simulink model "quadricopter"  (Simulink 7.4)
settings: Solver=ode45  StartTime=0.0  StopTime=2  RelTol=1e-5
values from neighbouring files (symbols this model uses):
  bm = 5106.8    [PID_init.m]    (also in quad_init.m)
  d = 0.16    [PID_init.m]    (also in quad_init.m)
  g = 9.8    [PID_init.m]    (also in quad_init.m)
  J_x = 7.8*10^-3    (= 0.0078)    [PID_init.m]    (also in quad_init.m)
  J_y = 7.8*10^-3    (= 0.0078)    [PID_init.m]    (also in quad_init.m)
  J_z = 10.22*10^-3    (= 0.01022)    [PID_init.m]    (also in quad_init.m)
  km = 342.4    [PID_init.m]    (also in quad_init.m)
  m = 0.835    [PID_init.m]    (also in quad_init.m)
libraries: aerolibtransform2 x1
settings Model: Creator=diogo  LastModifiedBy=diogo

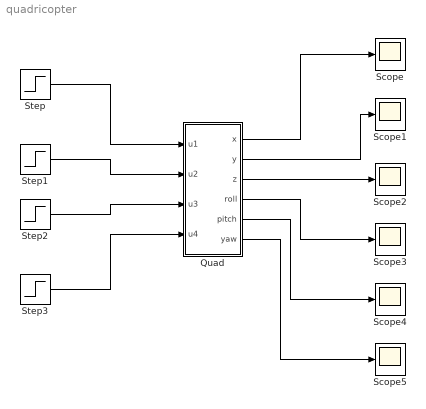
== system quadricopter ==
  Quad : Subsystem
  Scope{,1..5} (6 alike) : Scope
      Scope2 settings: TimeRange=0.03999999999999981  YMin=0  YMax=2e+223  SaveName=ScopeData2
      Scope3 settings: SaveName=ScopeData3
      Scope4 settings: SaveName=ScopeData4
      Scope5 settings: SaveName=ScopeData5
  Step{,1..3} (4 alike) : Step  Time=0  After=0.005  SampleTime=0
  wires:
  Quad/1(x) -> Scope/1
  Quad/2(y) -> Scope1/1
  Quad/3(z) -> Scope2/1
  Quad/4(roll) -> Scope3/1
  Quad/5(pitch) -> Scope4/1
  Quad/6(yaw) -> Scope5/1
  Step/1 -> Quad/1(u1)
  Step1/1 -> Quad/2(u2)
  Step2/1 -> Quad/3(u3)
  Step3/1 -> Quad/4(u4)

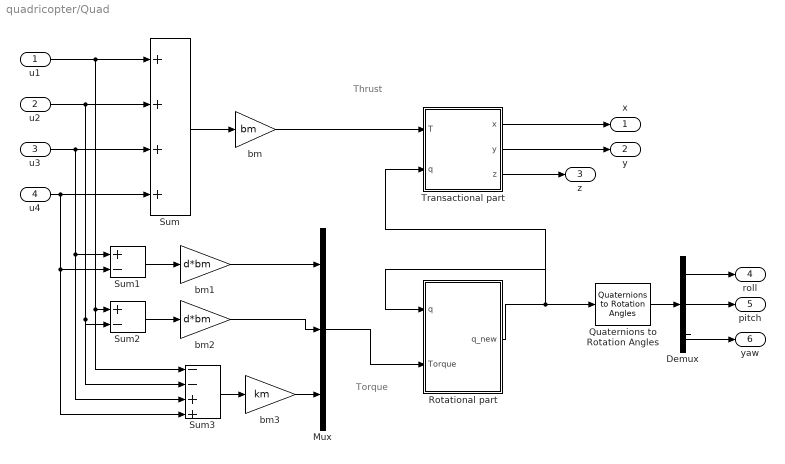
== system quadricopter/Quad ==
  note: Thrust
  note: Torque
  u1 : Inport  OutDataType=fixdt(1, 16)  OutScaling=2^0
  u2 : Inport  Port=2  OutDataType=fixdt(1, 16)  OutScaling=2^0
  u3 : Inport  Port=3  OutDataType=fixdt(1, 16)  OutScaling=2^0
  u4 : Inport  Port=4  OutDataType=fixdt(1, 16)  OutScaling=2^0
  Demux : Demux  Outputs=3
  Mux : Mux  Inputs=3
  Quaternions to Rotation Angles : aerolibtransform2/Quaternions to Rotation Angles  SystemSampleTime=-1  rotationOrder=XYZ
  Rotational part : Subsystem
  Sum : Sum  Inputs=++++  OutDataType=fixdt(1, 16)  OutScaling=2^0
  Sum1 : Sum  Inputs=+-  OutDataType=fixdt(1, 16)  OutScaling=2^0
  Sum2 : Sum  Inputs=+-  OutDataType=fixdt(1, 16)  OutScaling=2^0
  Sum3 : Sum  Inputs=--++  OutDataType=fixdt(1, 16)  OutScaling=2^0
  Transactional part : Subsystem
  bm : Gain  Gain=bm  ParameterDataType=fixdt(1, 16)  ParameterScaling=2^0  OutDataType=fixdt(1, 16)  OutScaling=2^0
  bm1 : Gain  Gain=d*bm  ParameterDataType=fixdt(1, 16)  ParameterScaling=2^0  OutDataType=fixdt(1, 16)  OutScaling=2^0
  bm2 : Gain  Gain=d*bm  ParameterDataType=fixdt(1, 16)  ParameterScaling=2^0  OutDataType=fixdt(1, 16)  OutScaling=2^0
  bm3 : Gain  Gain=km  ParameterDataType=fixdt(1, 16)  ParameterScaling=2^0  OutDataType=fixdt(1, 16)  OutScaling=2^0
  x : Outport  OutDataType=fixdt(1, 16)  OutScaling=2^0
  y : Outport  Port=2  OutDataType=fixdt(1, 16)  OutScaling=2^0
  z : Outport  Port=3  OutDataType=fixdt(1, 16)  OutScaling=2^0
  roll : Outport  Port=4  OutDataType=fixdt(1, 16)  OutScaling=2^0
  pitch : Outport  Port=5  OutDataType=fixdt(1, 16)  OutScaling=2^0
  yaw : Outport  Port=6  OutDataType=fixdt(1, 16)  OutScaling=2^0
  wires:
  u1/1 -> Sum/1, Sum2/1, Sum3/1
  u2/1 -> Sum/2, Sum2/2, Sum3/2
  u3/1 -> Sum/3, Sum1/1, Sum3/3
  u4/1 -> Sum/4, Sum1/2, Sum3/4
  Sum/1 -> bm/1
  bm/1 -> Transactional part/1(T)
  Transactional part/3(z) -> z/1
  Transactional part/2(y) -> y/1
  Transactional part/1(x) -> x/1
  Demux/1 -> roll/1
  Demux/2 -> pitch/1
  Demux/3 -> yaw/1
  Rotational part/1(q_new) -> Transactional part/2(q), Rotational part/1(q), Quaternions to Rotation Angles/1
  Sum1/1 -> bm1/1
  bm1/1 -> Mux/1
  Sum2/1 -> bm2/1
  bm2/1 -> Mux/2
  bm3/1 -> Mux/3
  Sum3/1 -> bm3/1
  Mux/1 -> Rotational part/2(Torque)
  Quaternions to Rotation Angles/1 -> Demux/1

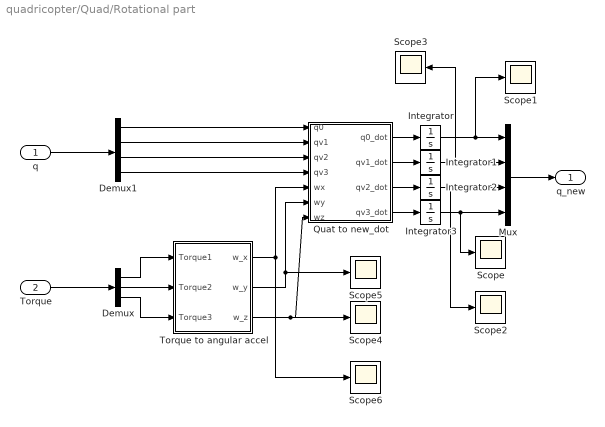
== system quadricopter/Quad/Rotational part ==
  q : Inport  OutDataType=fixdt(1, 16)  OutScaling=2^0
  Torque : Inport  Port=2  OutDataType=fixdt(1, 16)  OutScaling=2^0
  Demux : Demux  Outputs=3
  Demux1 : Demux
  Integrator : Integrator  InitialCondition=1
  Integrator1 : Integrator
  Integrator2 : Integrator
  Integrator3 : Integrator
  Mux : Mux
  Quat to new_dot : Subsystem
  Scope{,1..6} (7 alike) : Scope
      Scope settings: SaveName=ScopeData9
      Scope1 settings: SaveName=ScopeData10
      Scope2 settings: SaveName=ScopeData11
      Scope3 settings: SaveName=ScopeData12
      Scope4 settings: SaveName=ScopeData13
      Scope5 settings: SaveName=ScopeData14
      Scope6 settings: SaveName=ScopeData15
  Torque to angular accel : Subsystem
  q_new : Outport  OutDataType=fixdt(1, 16)  OutScaling=2^0
  wires:
  q/1 -> Demux1/1
  Demux1/1 -> Quat to new_dot/1(q0)
  Demux1/2 -> Quat to new_dot/2(qv1)
  Demux1/3 -> Quat to new_dot/3(qv2)
  Demux1/4 -> Quat to new_dot/4(qv3)
  Torque/1 -> Demux/1
  Demux/1 -> Torque to angular accel/1(Torque1)
  Demux/2 -> Torque to angular accel/2(Torque2)
  Demux/3 -> Torque to angular accel/3(Torque3)
  Torque to angular accel/1(w_x) -> Quat to new_dot/5(wx), Scope6/1
  Torque to angular accel/2(w_y) -> Quat to new_dot/6(wy), Scope5/1
  Torque to angular accel/3(w_z) -> Quat to new_dot/7(wz), Scope4/1
  Quat to new_dot/1(q0_dot) -> Integrator/1
  Quat to new_dot/2(qv1_dot) -> Integrator1/1
  Quat to new_dot/3(qv2_dot) -> Integrator2/1
  Quat to new_dot/4(qv3_dot) -> Integrator3/1
  Integrator/1 -> Mux/1, Scope1/1
  Integrator1/1 -> Mux/2, Scope3/1
  Integrator2/1 -> Mux/3, Scope2/1
  Integrator3/1 -> Mux/4, Scope/1
  Mux/1 -> q_new/1

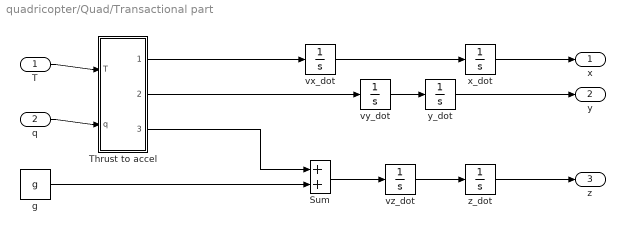
== system quadricopter/Quad/Transactional part ==
  T : Inport  OutDataType=fixdt(1, 16)  OutScaling=2^0
  q : Inport  Port=2  OutDataType=fixdt(1, 16)  OutScaling=2^0
  Sum : Sum  OutDataType=fixdt(1, 16)  OutScaling=2^0
  Thrust to accel : Subsystem
  g : Constant  Value=g  OutDataType=fixdt(1, 16)  OutScaling=2^0
  vx_dot : Integrator
  vy_dot : Integrator
  vz_dot : Integrator
  x_dot : Integrator
  y_dot : Integrator
  z_dot : Integrator
  x : Outport  OutDataType=fixdt(1, 16)  OutScaling=2^0
  y : Outport  Port=2  OutDataType=fixdt(1, 16)  OutScaling=2^0
  z : Outport  Port=3  OutDataType=fixdt(1, 16)  OutScaling=2^0
  wires:
  x_dot/1 -> x/1
  y_dot/1 -> y/1
  z_dot/1 -> z/1
  g/1 -> Sum/2
  T/1 -> Thrust to accel/1(T)
  q/1 -> Thrust to accel/2(q)
  Thrust to accel/1(vx_dot) -> vx_dot/1
  Thrust to accel/2(vy_dot) -> vy_dot/1
  Thrust to accel/3(vz_dot) -> Sum/1
  vz_dot/1 -> z_dot/1
  vy_dot/1 -> y_dot/1
  vx_dot/1 -> x_dot/1
  Sum/1 -> vz_dot/1

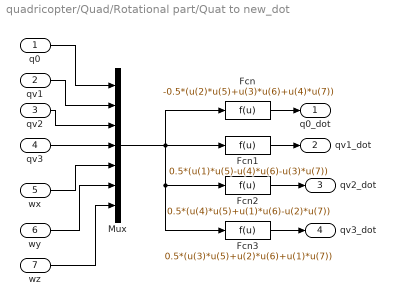
== system quadricopter/Quad/Rotational part/Quat to new_dot ==
  q0 : Inport  OutDataType=fixdt(1, 16)  OutScaling=2^0
  qv1 : Inport  Port=2  OutDataType=fixdt(1, 16)  OutScaling=2^0
  qv2 : Inport  Port=3  OutDataType=fixdt(1, 16)  OutScaling=2^0
  qv3 : Inport  Port=4  OutDataType=fixdt(1, 16)  OutScaling=2^0
  wx : Inport  Port=5  OutDataType=fixdt(1, 16)  OutScaling=2^0
  wy : Inport  Port=6  OutDataType=fixdt(1, 16)  OutScaling=2^0
  wz : Inport  Port=7  OutDataType=fixdt(1, 16)  OutScaling=2^0
  Fcn : Fcn  Expr=-0.5*(u(2)*u(5)+u(3)*u(6)+u(4)*u(7))
  Fcn1 : Fcn  Expr=0.5*(u(1)*u(5)-u(4)*u(6)-u(3)*u(7))
  Fcn2 : Fcn  Expr=0.5*(u(4)*u(5)+u(1)*u(6)-u(2)*u(7))
  Fcn3 : Fcn  Expr=0.5*(u(3)*u(5)+u(2)*u(6)+u(1)*u(7))
  Mux : Mux  Inputs=7
  q0_dot : Outport  OutDataType=fixdt(1, 16)  OutScaling=2^0
  qv1_dot : Outport  Port=2  OutDataType=fixdt(1, 16)  OutScaling=2^0
  qv2_dot : Outport  Port=3  OutDataType=fixdt(1, 16)  OutScaling=2^0
  qv3_dot : Outport  Port=4  OutDataType=fixdt(1, 16)  OutScaling=2^0
  wires:
  q0/1 -> Mux/1
  qv1/1 -> Mux/2
  qv2/1 -> Mux/3
  qv3/1 -> Mux/4
  wx/1 -> Mux/5
  wy/1 -> Mux/6
  wz/1 -> Mux/7
  Mux/1 -> Fcn/1, Fcn1/1, Fcn2/1, Fcn3/1
  Fcn/1 -> q0_dot/1
  Fcn1/1 -> qv1_dot/1
  Fcn2/1 -> qv2_dot/1
  Fcn3/1 -> qv3_dot/1

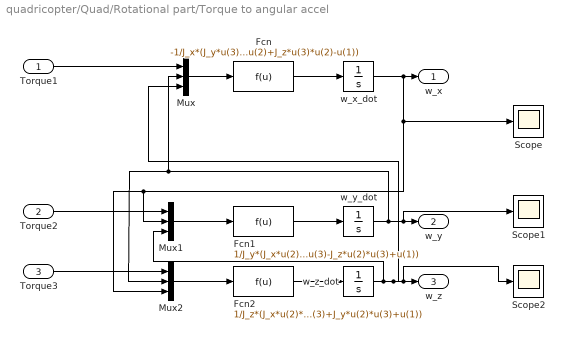
== system quadricopter/Quad/Rotational part/Torque to angular accel ==
  Torque1 : Inport  OutDataType=fixdt(1, 16)  OutScaling=2^0
  Torque2 : Inport  Port=2  OutDataType=fixdt(1, 16)  OutScaling=2^0
  Torque3 : Inport  Port=3  OutDataType=fixdt(1, 16)  OutScaling=2^0
  Fcn : Fcn  Expr=-1/J_x*(J_y*u(3)*u(2)+J_z*u(3)*u(2)-u(1))
  Fcn1 : Fcn  Expr=1/J_y*(J_x*u(2)*u(3)-J_z*u(2)*u(3)+u(1))
  Fcn2 : Fcn  Expr=1/J_z*(J_x*u(2)*u(3)+J_y*u(2)*u(3)+u(1))
  Mux : Mux  Inputs=3
  Mux1 : Mux  Inputs=3
  Mux2 : Mux  Inputs=3
  Scope : Scope
      settings: SaveName=ScopeData6
  Scope1 : Scope
      settings: SaveName=ScopeData7
  Scope2 : Scope
      settings: SaveName=ScopeData8
  w_x_dot : Integrator
  w_y_dot : Integrator
  w_z_dot : Integrator
  w_x : Outport  OutDataType=fixdt(1, 16)  OutScaling=2^0
  w_y : Outport  Port=2  OutDataType=fixdt(1, 16)  OutScaling=2^0
  w_z : Outport  Port=3  OutDataType=fixdt(1, 16)  OutScaling=2^0
  wires:
  w_x_dot/1 -> w_x/1, Mux1/2, Mux2/3, Scope/1
  w_y_dot/1 -> Mux/2, Mux2/2, w_y/1, Scope1/1
  w_z_dot/1 -> Mux/3, w_z/1, Scope2/1, Mux1/3
  Torque1/1 -> Mux/1
  Mux/1 -> Fcn/1
  Fcn/1 -> w_x_dot/1
  Torque2/1 -> Mux1/1
  Mux1/1 -> Fcn1/1
  Fcn1/1 -> w_y_dot/1
  Fcn2/1 -> w_z_dot/1
  Torque3/1 -> Mux2/1
  Mux2/1 -> Fcn2/1

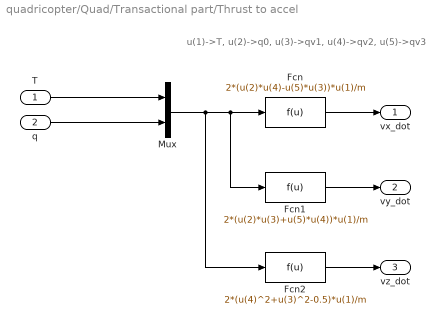
== system quadricopter/Quad/Transactional part/Thrust to accel ==
  note: u(1)->T, u(2)->q0, u(3)->qv1, u(4)->qv2, u(5)->qv3
  T : Inport  OutDataType=fixdt(1, 16)  OutScaling=2^0
  q : Inport  Port=2  OutDataType=fixdt(1, 16)  OutScaling=2^0
  Fcn : Fcn  Expr=2*(u(2)*u(4)-u(5)*u(3))*u(1)/m
  Fcn1 : Fcn  Expr=2*(u(2)*u(3)+u(5)*u(4))*u(1)/m
  Fcn2 : Fcn  Expr=2*(u(4)^2+u(3)^2-0.5)*u(1)/m
  Mux : Mux  Inputs=2
  vx_dot : Outport  OutDataType=fixdt(1, 16)  OutScaling=2^0
  vy_dot : Outport  Port=2  OutDataType=fixdt(1, 16)  OutScaling=2^0
  vz_dot : Outport  Port=3  OutDataType=fixdt(1, 16)  OutScaling=2^0
  wires:
  T/1 -> Mux/1
  q/1 -> Mux/2
  Mux/1 -> Fcn/1, Fcn1/1, Fcn2/1
  Fcn/1 -> vx_dot/1
  Fcn1/1 -> vy_dot/1
  Fcn2/1 -> vz_dot/1
